simulink model "analog_model_power_v13"  (R2015a)
settings: Solver=ode45  StartTime=0.0  StopTime=12e-3  MaxStep=1e-6  RelTol=1e-3
StartFcn:
  | R1
  | R2
  | R3
  | R4
  | C1
values from neighbouring files (symbols this model uses):
  C = Kp + Ki/s + Kd*s    [DC_Motor_Speed_Digital_Controller_Design_example.m]    (also in GalvoModel_v3_discret_proc.m = gv.tfCCv2p2; InvertedPendulum.m = [1 0 0 0; gtktermFun1.m = textscan(fd, ')
  C2 = 100e-12    (= 1e-10)    [Galvo_sys_proto_v13_OFFSETS_MODEL_PT1B_OLDproc.m]    (also in Galvo_sys_proto_v13_OFFSETS_MODEL_PT1B_proc.m = 1e-11)
  R1 = 1.2e3    (= 1200)    [GalvoModel_v6_sys.m]    (also in Galvo_process_analyze.m = 10000; Galvo_sys_proto_v13_OFFSETS_MODEL_PT1B_OLDproc.m = 5000; Galvo_sys_proto_v13_OFFSETS_MODEL_PT1B_proc.m = 5100; frequenzgang_nichtinvert_opamp_koblitz_eas.m = 0.015)
  R2 = 20e3    (= 20000)    [Galvo_process_analyze.m]    (also in Galvo_sys_proto_v13_OFFSETS_MODEL_PT1B_OLDproc.m = 45000; Galvo_sys_proto_v13_OFFSETS_MODEL_PT1B_proc.m = (Kp-1)*R1; frequenzgang_nichtinvert_opamp_koblitz_eas.m = RL+j*w*L)
  R3 = 1e3    (= 1000)    [Galvo_sys_proto_v13_OFFSETS_MODEL_PT1B_OLDproc.m]    (also in Galvo_sys_proto_v13_OFFSETS_MODEL_PT1B_proc.m = 1e+33)
  R4 = R1    (= 3300)    [Galvo_sys_proto_v13_OFFSETS_MODEL_PT1B_proc.m]    (also in OpAmp_addierer_spannTeiler.m = 10)
  s = tf('s')    [DC_Motor_Speed_Digital_Controller_Design_example.m]    (also in GalvoBIGMatlab_cortex_Link.m = instrfind; GalvoMatlab_cortex_Link.m = MdbOpenPort(); GalvoModel_v6_sys.m; Galvo_process_analyze.m = struct)
undefined symbols (not defined in the file or in its folder): Z4
libraries: fl_lib x24, nesl_utility x6, elec_lib x3, slctrlblks x2, simulink x2
settings Model: Creator=mainster  LastModifiedBy=mainster
settings DebuggingCC: UnderspecifiedInitializationDetection=Classic  MergeDetectMultiDrivingBlocksExec=none  SolverPrmCheckMsg=warning  StateNameClashWarn=warning

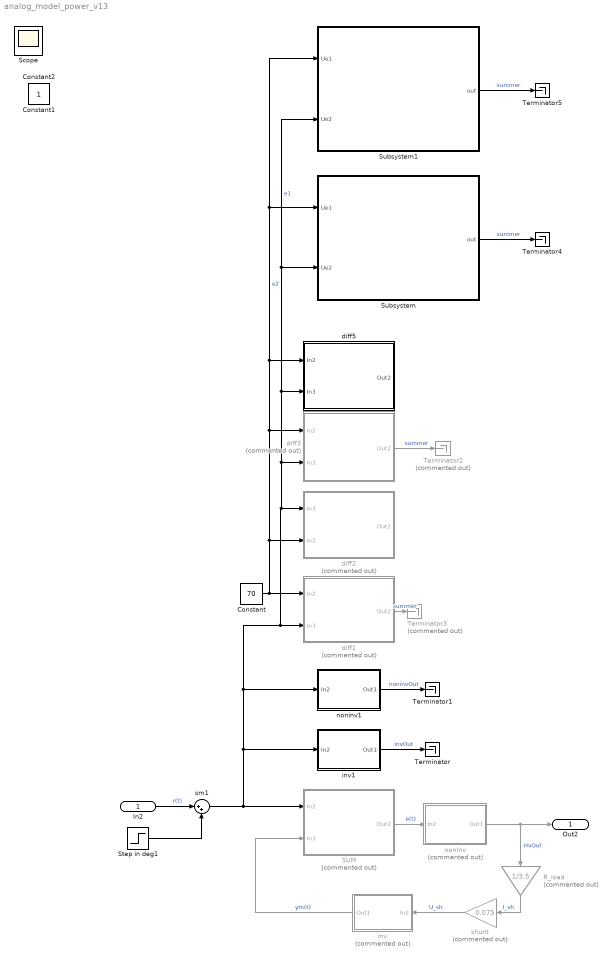
== system analog_model_power_v13 ==
  In2 : Inport
  Constant : Constant  Value=70
  R_load : Gain  Commented=on  Gain=1/3.5
  SUM : Subsystem  Commented=on  mask{R1=3.3e3, R2=3.3e3, R3=3.3e3, R4=3.3e3, C1=1e-12}
      mask prompts: R1 "Value for R1"; R2 "Value for R2"; R3 "Value for R3"; R4 "Value for R4"; C1 "Value for C1"
      mask Display: fprintf('R1=%gohm\nR2=%gohm\nR3=%gohm\nR4=%gohm\nC1=%gnF\n',R1,R2,R3,R4,C1*1e9)
  Step in deg1 : Step  Time=1e-3  SampleTime=0  ZeroCross=off
      settings: AttributesFormatString=Ampl.: %<After>\ntime:%<Time>
  Subsystem : Subsystem  mask{R1=3.3e3, R2=3.3e3, R3=3.3e3, R4=3.3e3}
      mask prompts: R1 "Enter R1"; R2 "Enter R2"; R3 "Enter R3"; R4 "Enter R4"
      mask Display:
      | image(imread('/media/storage/data_notebook/HS_Karlsruhe/xy_galvoscanner/gewichteter_Diff.png'));
      | text(.71, .65, num2str(R4))
      | text(.26, .675, num2str(R3))
      | text(.26, .265, num2str(R1))
      | text(.46, .045, num2str(R2))
  Subsystem1 : Subsystem  mask{R1=3.3e3, R2=3.3e3, R3=3.3e3, R4=3.3e3, C1=100e-12}
      mask prompts: R1 "Enter R1"; R2 "Enter R2"; R3 "Enter R3"; R4 "Enter R4"; C1 "Enter C1"
      mask Callback R4:
      | if C1>0
      |     Z4=R4/(1+s*C1*R4)
      | end
      mask Callback C1:
      | if R4>0
      |     Z4=R4/(1+s*C1*R4)
      | end
      mask Display:
      | image(imread('/media/storage/data_notebook/HS_Karlsruhe/xy_galvoscanner/gewichteter_Diff_lead.png'));
      | text(.71, .65, num2str(R4))
      | text(.26, .675, num2str(R3))
      | text(.26, .265, num2str(R1))
      | text(.46, .045, num2str(R2))
      | text(.76, .842, num2str(R4))
  Terminator{,1,4..5} (4 alike) : Terminator
  Terminator2 : Terminator  Commented=on
  Terminator3 : Terminator  Commented=on
  diff1 : Subsystem  Commented=on  mask{R1=3.3e3, R2=3.3e3, R3=3.3e3, R4=3.3e3, C1=1e-08}
      mask prompts: R1 "Value for R1"; R2 "Value for R2"; R3 "Value for R3"; R4 "Value for R4"; C1 "Value for C1"
      mask Display:
      | fprintf('R1=%gohm\nR2=%gohm\nR3=%gohm\nR4=%gohm\nC1=%gnF\n',R1,R2,R3,R4,C1*1e9)
      | % port_label('input',1,'Ue1');
      | % port_label('input',2,'Ue2');
  diff2 : Subsystem  Commented=on  mask{R1=3.3e3, R2=3.3e3, R3=3.3e3, R4=3.3e3, C1=1e-11}
      mask prompts: R1 "Value for R1"; R2 "Value for R2"; R3 "Value for R3"; R4 "Value for R4"; C1 "Value for C1"
      mask Display:
      | fprintf('R1=%gohm\nR2=%gohm\nR3=%gohm\nR4=%gohm\nC1=%gnF\n',R1,R2,R3,R4,C1*1e9)
      | % port_label('input',1,'Ue1');
      | % port_label('input',2,'Ue2');
  diff3 : Subsystem  Commented=on  mask{R1=3e3, gR1=1/R1, R2=3e3, gR2=1/R2, R3=3e3, R4=3e3, R4R3=R4/R3, C1=1e-11, gC1=0, C2=1e-35, gC2=1/C2}
      mask prompts: R1 "Value for R1"; gR1 "Gain:"; R2 "Value for R2"; gR2 "Gain:"; R3 "Value for R3"; R4 "Value for R4"; R4R3 "Gain:"; C1 "Value for C1"; C2 "Value for C2"; gC2 "Gain:"
      mask Callback R1: gR1=1/R1
      mask TypeOptions gR1: Gain3/Gain
      mask Callback R2: gR2=1/R2
      mask TypeOptions gR2: Gain1/Gain
      mask Callback R3:
      | if R3>0
      |     R4R3 = R4/R3;
      | end
      mask Callback R4:
      | if R3>0
      |     R4R3 = R4/R3;
      | end
      mask TypeOptions R4R3: Gain4/Gain
      mask Callback C1: gC1=1/C1
      mask Callback C2: gC2=1/C2
      mask TypeOptions gC2: Gain/Gain
      mask Display:
      | fprintf('R1=%gohm\nR2=%gohm\nR3=%gohm\nR4=%gohm\nC1=%gF\nC2=%gF\n',R1,R2,R3,R4,C1,C2)
      | % port_label('input',1,'Ue1');
      | % port_label('input',2,'Ue2');
  diff5 : Subsystem  mask{R1=3.3e3, R2=3.3e3, R3=3.3e3, R4=3.3e3, C1=1e-11, C2=1}
      mask prompts: R1 "Value for R1"; R2 "Value for R2"; R3 "Value for R3"; R4 "Value for R4"; C1 "Value for C1"; C2 "Value for C2"
      mask Display:
      | fprintf('R1=%gohm\nR2=%gohm\nR3=%gohm\nR4=%gohm\nC1=%gnF\n',R1,R2,R3,R4,C1*1e9)
      | % port_label('input',1,'Ue1');
      | % port_label('input',2,'Ue2');
  inv : Subsystem  Commented=on  mask{R1=27, R2=270, C1=1}
      mask prompts: R1 "Value for R1"; R2 "Value for R2"; C1 "Value for C1"
      mask Display: fprintf('R1=%gohm\nR2=%gohm\nC1=%gnF\n',R1,R2,C1*1e9)
  inv1 : Subsystem  mask{R1=1e3, R2=10e3, C2=1e-11}
      mask prompts: R1 "Value for R1"; R2 "Value for R2"; C2 "Value for C2"
      mask Display: fprintf('R1=%gohm\nR2=%gohm\nC2=%gF\n',R1,R2,C2)
  nonInv : Subsystem  Commented=on  mask{R1=5.1e3, R2=2*5.1e3, C2=1e-08}
      mask prompts: R1 "Value for R1"; R2 "Value for R2"; C2 "Value for C2"
      mask Display: fprintf('R1=%gohm\nR2=%gohm\nC1=C2=%gF\n',R1,R2,C2)
  noninv1 : Subsystem  mask{R1=1e3, R2=9e3, C2=1e-08}
      mask prompts: R1 "Value for R1"; R2 "Value for R2"; C2 "Value for C2"
      mask Display: fprintf('R1=%gohm\nR2=%gohm\nC2=%gF\n',R1,R2,C2)
  shunt : Gain  Commented=on  Gain=0.075
  sm1 : Sum  Inputs=|++
  Out2 : Outport
  Constant1 : Constant  IOType=siggen
  Constant2 : Constant  IOType=siggen
  Scope : Scope  NumInputPorts=4
      settings: ShowLegends=on  TimeRange=0.012  YMin=-5~-5~-5~-5  YMax=5~5~5~5  MaxDataPoints=7500
  wires:
  SUM/1(Out2) -> nonInv/1(In2)  "e(t)"
  In2/1 -> sm1/1  "r(t)"
  inv/1(Out1) -> SUM/2(In3)  "ym(t)"
  nonInv/1(Out1) -> R_load/1, Out2/1  "HvOut"
  R_load/1 -> shunt/1  "I_sh"
  shunt/1 -> inv/1(In2)  "U_sh"
  Step in deg1/1 -> sm1/2
  inv1/1(Out1) -> Terminator/1  "invOut"
  noninv1/1(Out1) -> Terminator1/1  "noninvOut"
  diff3/1(Out2) -> Terminator2/1  "summer"
  diff1/1(Out2) -> Terminator3/1  "summer"
  Subsystem/1(out) -> Terminator4/1  "summer"
  sm1/1 -> Subsystem1/2(Ue2), Subsystem/2(Ue2), diff5/2(In3), diff3/2(In3), diff2/1(In3), diff1/2(In3), noninv1/1(In2), inv1/1(In2), SUM/1(In2)  "e1"
  Constant/1 -> Subsystem1/1(Ue1), Subsystem/1(Ue1), diff5/1(In2), diff3/1(In2), diff2/2(In2), diff1/1(In2)  "e2"
  Subsystem1/1(out) -> Terminator5/1  "summer"

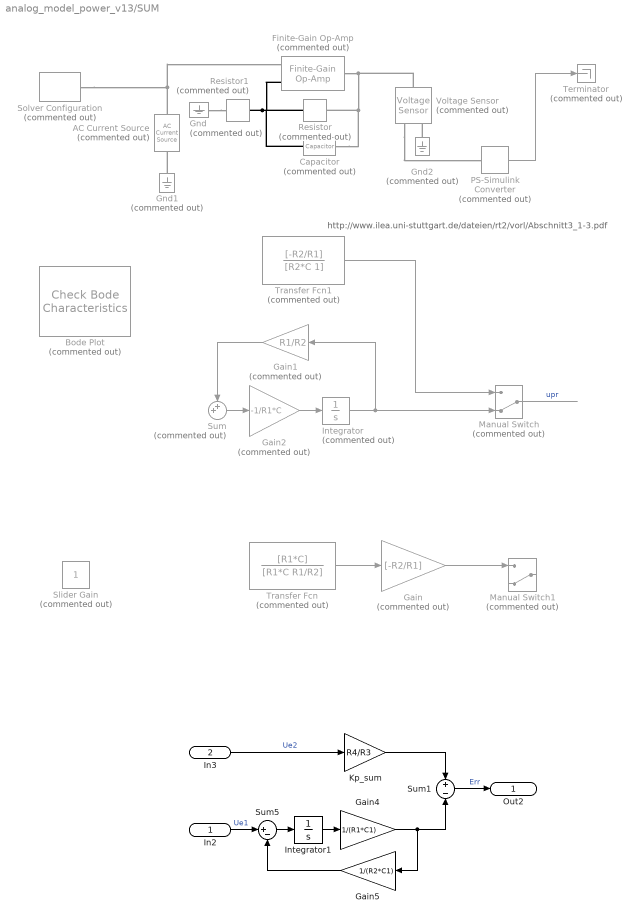
== system analog_model_power_v13/SUM ==
  note: http://www.ilea.uni-stuttgart.de/dateien/rt2/vorl/Abschnitt3_1-3.pdf
  In2 : Inport
  In3 : Inport  Port=2
  AC Current Source : fl_lib/Electrical/Electrical Sources/AC Current Source  Commented=on  amp=1 A  shift=0 deg  frequency=1000 Hz  omega=0 rad/s  i_Log=off  v_Log=off  LocalVarNames=|i|v  LocalVarDescs=|i|v  LocalVarLogging=[0 0]
  Bode Plot : slctrlblks/Model Verification/Check Bode  Characteristics  Commented=on  InstantiateOnLoad=on  SaveOperatingPoints=off  LinearizationIOs={'/Gcc(s)/sub1/In1', 1, 'in', 'off', '';'/Gcc(s)/sub1/Gain', 1, 'out', 'on', '';'/Gcc(s)/sub1/Manual Switch', 1, 'out', 'on', '';'/Gcc(s)/sub1/Manual Switch1', 1, 'out', 'on', ''}  LinearizeAt=SnapshotTimes  SnapshotTimes=[0]  TriggerType=rising  SampleTime=auto  RateConversionMethod=zoh  PreWarpFreq=10  UseExactDelayModel=off  UseFullBlockNameLabels=off  UseBusSignalLabels=off  enabled=on  stopWhenAssertionFail=off  export=off  ViewDlgPos=[100 200 510 390]  OpenViewOnLoad=off  LaunchViewOnOpen=on  FrequencyUnits=rad/s  MagnitudeUnits=dB  PhaseUnits=deg  TimeUnits=seconds  EnableUpperBound=off  UpperBoundFrequencies=[]  UpperBoundMagnitudes=[]  EnableLowerBound=off  LowerBoundFrequencies=[]  LowerBoundMagnitudes=[]
  Capacitor : fl_lib/Electrical/Electrical Elements/Capacitor  Commented=on  c=1e-6 F  v0=0 V  r=1e-6 Ohm  g=0 1/Ohm  i_Log=off  v_Log=off  vc_Log=off  LocalVarNames=|i|v|vc  LocalVarDescs=|i|v|Internal variable for voltage across capacitor term  LocalVarLogging=[0 0 0]
  Finite-Gain Op-Amp : elec_lib/Integrated Circuits/Finite-Gain Op-Amp  Commented=on  A=1000  Rin=1e+6 Ohm  Rout=100 Ohm  Vmin=-15 V  Vmax=15 V  LocalVarLogging=[]
  Gain : Gain  Commented=on  Gain=[-R2/R1]
  Gain1 : Gain  Commented=on  Gain=R1/R2
  Gain2 : Gain  Commented=on  Gain=-1/R1*C
  Gain4 : Gain  Gain=1/(R1*C1)
  Gain5 : Gain  Gain=1/(R2*C1)
  Gnd : fl_lib/Electrical/Electrical Elements/Electrical Reference  Commented=on  i_Log=off  LocalVarNames=|i  LocalVarDescs=|i  LocalVarLogging=0
  Gnd1 : fl_lib/Electrical/Electrical Elements/Electrical Reference  Commented=on  i_Log=off  LocalVarNames=|i  LocalVarDescs=|i  LocalVarLogging=0
  Gnd2 : fl_lib/Electrical/Electrical Elements/Electrical Reference  Commented=on  i_Log=off  LocalVarNames=|i  LocalVarDescs=|i  LocalVarLogging=0
  Integrator : Integrator  Commented=on
  Integrator1 : Integrator
  Kp_sum : Gain  Gain=R4/R3
  Manual Switch : ManualSwitch  Commented=on  CurrentSetting=0
  Manual Switch1 : ManualSwitch  Commented=on  CurrentSetting=0
  PS-Simulink Converter : nesl_utility/PS-Simulink Converter  Commented=on  PhysicalDomain=network_engine_domain  SubClassName=ps_output  LeftPortType=input  RightPortType=output  PseudoPeriodic=off  Frequencies=[]  Unit=1  AffineConversion=off
  Resistor : fl_lib/Electrical/Electrical Elements/Resistor  Commented=on  R=R2 Ohm  i_Log=off  v_Log=off  LocalVarNames=|i|v  LocalVarDescs=|i|v  LocalVarLogging=[0 0]
      settings: AttributesFormatString=%<R>
  Resistor1 : fl_lib/Electrical/Electrical Elements/Resistor  Commented=on  R=R1 Ohm  i_Log=off  v_Log=off  LocalVarNames=|i|v  LocalVarDescs=|i|v  LocalVarLogging=[0 0]
      settings: AttributesFormatString=%<R>
  Slider Gain : simulink/Math Operations/Slider Gain  Commented=on  low=0  gain=1  high=2
  Solver Configuration : nesl_utility/Solver Configuration  Commented=on  PhysicalDomain=network_engine_domain  SubClassName=solver  LeftPortType=input  RightPortType=generic  Accelerate=off  Tones=[]  Harmonics=[]  SimulateNoise=off  Profile=off  UseLocalSampling=off  EnableSwitchedLinearOptims=on  FrequencyDomain=off  UseCCode=off  UseNewInitialization=off  DoDC=off  ResidualTolerance=1e-09  UseLocalSolver=off  LocalSolverChoice=NE_BACKWARD_EULER_ADVANCER  LocalSolverSampleTime=0.001  DoFixedCost=off  MaxNonlinIter=3  MaxModeIter=2  LinearAlgebra=Sparse  DelaysMemoryBudget=1024
  Sum : Sum  Commented=on  Inputs=++|
  Sum1 : Sum  Inputs=+|-
  Sum5 : Sum  Inputs=|+-
  Terminator : Terminator  Commented=on
  Transfer Fcn : TransferFcn  Commented=on  Numerator=[R1*C]  Denominator=[R1*C R1/R2]
  Transfer Fcn1 : TransferFcn  Commented=on  Numerator=[-R2/R1]  Denominator=[R2*C 1]
  Voltage Sensor : fl_lib/Electrical/Electrical Sensors/Voltage Sensor  Commented=on  i1_Log=off  v1_Log=off  LocalVarNames=|i1|v1  LocalVarDescs=|i1|v1  LocalVarLogging=[0 0]
  Out2 : Outport
  wires:
  Integrator1/1 -> Gain4/1
  Gain4/1 -> Gain5/1, Sum1/2
  ? -> Transfer Fcn/1, Transfer Fcn1/1, Sum/2
  Transfer Fcn/1 -> Gain/1
  Sum5/1 -> Integrator1/1
  Manual Switch/1 -> ?  "upr"
  Gain/1 -> Manual Switch1/1
  Gain1/1 -> Sum/1
  Integrator/1 -> Gain1/1, Manual Switch/2
  Sum/1 -> Gain2/1
  Gain2/1 -> Integrator/1
  Transfer Fcn1/1 -> Manual Switch/1
  PS-Simulink Converter/1 -> Terminator/1
  Gain5/1 -> Sum5/2
  In3/1 -> Kp_sum/1  "Ue2"
  Kp_sum/1 -> Sum1/1
  In2/1 -> Sum5/1  "Ue1"
  Sum1/1 -> Out2/1  "Err"
  connections:
  Resistor1/RConn1 -- Capacitor/LConn1 -- Finite-Gain Op-Amp/LConn2 -- Resistor/LConn1
  Solver Configuration/RConn1 -- Finite-Gain Op-Amp/LConn1 -- AC Current Source/LConn1
  Gnd1/LConn1 -- AC Current Source/RConn1
  Voltage Sensor/RConn1 -- PS-Simulink Converter/LConn1
  Gnd2/LConn1 -- Voltage Sensor/RConn2
  Gnd/LConn1 -- Resistor1/LConn1
  Voltage Sensor/LConn1 -- Capacitor/RConn1 -- Resistor/RConn1 -- Finite-Gain Op-Amp/RConn1

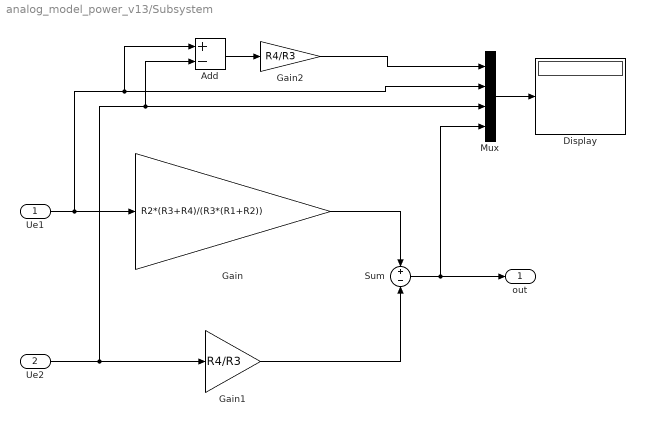
== system analog_model_power_v13/Subsystem ==
  Ue1 : Inport
  Ue2 : Inport  Port=2
  Add : Sum  Inputs=+-
  Display : Display
  Gain : Gain  Gain=R2*(R3+R4)/(R3*(R1+R2))
  Gain1 : Gain  Gain=R4/R3
  Gain2 : Gain  Gain=R4/R3
  Mux : Mux
  Sum : Sum  Inputs=+|-
  out : Outport
  wires:
  Gain/1 -> Sum/1
  Gain1/1 -> Sum/2
  Ue1/1 -> Mux/2, Add/1, Gain/1
  Ue2/1 -> Mux/3, Add/2, Gain1/1
  Sum/1 -> Mux/4, out/1
  Mux/1 -> Display/1
  Add/1 -> Gain2/1
  Gain2/1 -> Mux/1

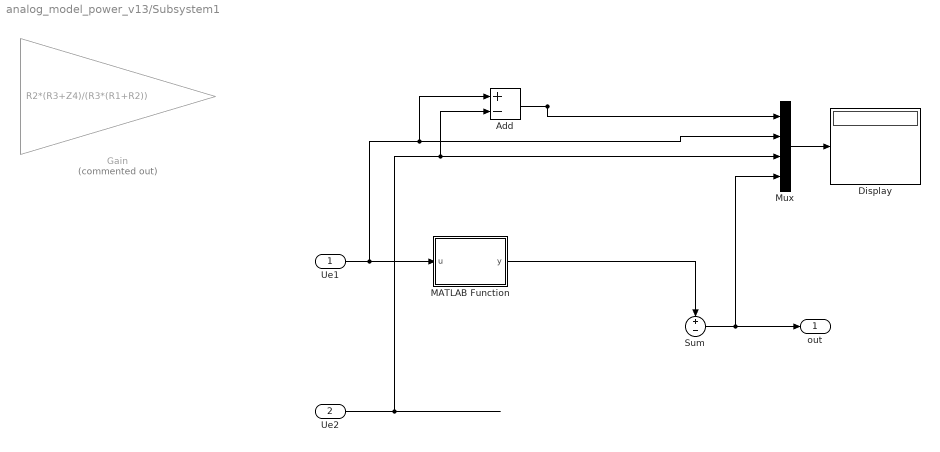
== system analog_model_power_v13/Subsystem1 ==
  Ue1 : Inport
  Ue2 : Inport  Port=2
  Add : Sum  Inputs=+-
  Display : Display
  Gain : Gain  Commented=on  Gain=R2*(R3+Z4)/(R3*(R1+R2))
  MATLAB Function : MATLAB Function  TreatAsAtomicUnit=on
  Mux : Mux
  Sum : Sum  Inputs=+|-
  out : Outport
  wires:
  MATLAB Function/1(y) -> Sum/1
  ? -> Sum/2
  Ue1/1 -> MATLAB Function/1(u), Mux/2, Add/1
  Ue2/1 -> Mux/3, Add/2
  Sum/1 -> Mux/4, out/1
  Mux/1 -> Display/1
  Add/1 -> Mux/1

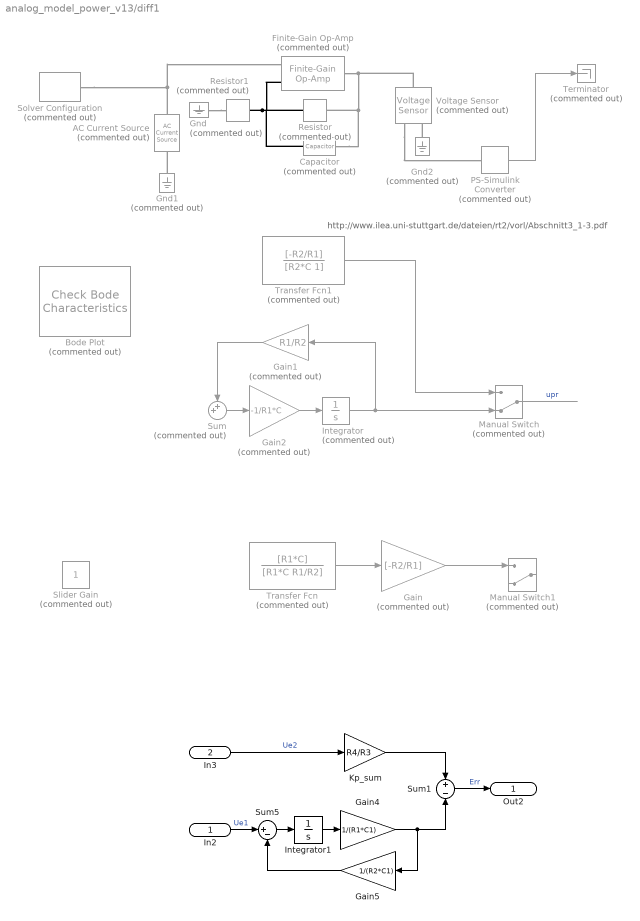
== system analog_model_power_v13/diff1 ==
  note: http://www.ilea.uni-stuttgart.de/dateien/rt2/vorl/Abschnitt3_1-3.pdf
  In2 : Inport
  In3 : Inport  Port=2
  AC Current Source : fl_lib/Electrical/Electrical Sources/AC Current Source  Commented=on  amp=1 A  shift=0 deg  frequency=1000 Hz  omega=0 rad/s  i_Log=off  v_Log=off  LocalVarNames=|i|v  LocalVarDescs=|i|v  LocalVarLogging=[0 0]
  Bode Plot : slctrlblks/Model Verification/Check Bode  Characteristics  Commented=on  InstantiateOnLoad=on  SaveOperatingPoints=off  LinearizationIOs={'/Gcc(s)/sub1/In1', 1, 'in', 'off', '';'/Gcc(s)/sub1/Gain', 1, 'out', 'on', '';'/Gcc(s)/sub1/Manual Switch', 1, 'out', 'on', '';'/Gcc(s)/sub1/Manual Switch1', 1, 'out', 'on', ''}  LinearizeAt=SnapshotTimes  SnapshotTimes=[0]  TriggerType=rising  SampleTime=auto  RateConversionMethod=zoh  PreWarpFreq=10  UseExactDelayModel=off  UseFullBlockNameLabels=off  UseBusSignalLabels=off  enabled=on  stopWhenAssertionFail=off  export=off  ViewDlgPos=[100 200 510 390]  OpenViewOnLoad=off  LaunchViewOnOpen=on  FrequencyUnits=rad/s  MagnitudeUnits=dB  PhaseUnits=deg  TimeUnits=seconds  EnableUpperBound=off  UpperBoundFrequencies=[]  UpperBoundMagnitudes=[]  EnableLowerBound=off  LowerBoundFrequencies=[]  LowerBoundMagnitudes=[]
  Capacitor : fl_lib/Electrical/Electrical Elements/Capacitor  Commented=on  c=1e-6 F  v0=0 V  r=1e-6 Ohm  g=0 1/Ohm  i_Log=off  v_Log=off  vc_Log=off  LocalVarNames=|i|v|vc  LocalVarDescs=|i|v|Internal variable for voltage across capacitor term  LocalVarLogging=[0 0 0]
  Finite-Gain Op-Amp : elec_lib/Integrated Circuits/Finite-Gain Op-Amp  Commented=on  A=1000  Rin=1e+6 Ohm  Rout=100 Ohm  Vmin=-15 V  Vmax=15 V  LocalVarLogging=[]
  Gain : Gain  Commented=on  Gain=[-R2/R1]
  Gain1 : Gain  Commented=on  Gain=R1/R2
  Gain2 : Gain  Commented=on  Gain=-1/R1*C
  Gain4 : Gain  Gain=1/(R1*C1)
  Gain5 : Gain  Gain=1/(R2*C1)
  Gnd : fl_lib/Electrical/Electrical Elements/Electrical Reference  Commented=on  i_Log=off  LocalVarNames=|i  LocalVarDescs=|i  LocalVarLogging=0
  Gnd1 : fl_lib/Electrical/Electrical Elements/Electrical Reference  Commented=on  i_Log=off  LocalVarNames=|i  LocalVarDescs=|i  LocalVarLogging=0
  Gnd2 : fl_lib/Electrical/Electrical Elements/Electrical Reference  Commented=on  i_Log=off  LocalVarNames=|i  LocalVarDescs=|i  LocalVarLogging=0
  Integrator : Integrator  Commented=on
  Integrator1 : Integrator
  Kp_sum : Gain  Gain=R4/R3
  Manual Switch : ManualSwitch  Commented=on  CurrentSetting=0
  Manual Switch1 : ManualSwitch  Commented=on  CurrentSetting=0
  PS-Simulink Converter : nesl_utility/PS-Simulink Converter  Commented=on  PhysicalDomain=network_engine_domain  SubClassName=ps_output  LeftPortType=input  RightPortType=output  PseudoPeriodic=off  Frequencies=[]  Unit=1  AffineConversion=off
  Resistor : fl_lib/Electrical/Electrical Elements/Resistor  Commented=on  R=R2 Ohm  i_Log=off  v_Log=off  LocalVarNames=|i|v  LocalVarDescs=|i|v  LocalVarLogging=[0 0]
      settings: AttributesFormatString=%<R>
  Resistor1 : fl_lib/Electrical/Electrical Elements/Resistor  Commented=on  R=R1 Ohm  i_Log=off  v_Log=off  LocalVarNames=|i|v  LocalVarDescs=|i|v  LocalVarLogging=[0 0]
      settings: AttributesFormatString=%<R>
  Slider Gain : simulink/Math Operations/Slider Gain  Commented=on  low=0  gain=1  high=2
  Solver Configuration : nesl_utility/Solver Configuration  Commented=on  PhysicalDomain=network_engine_domain  SubClassName=solver  LeftPortType=input  RightPortType=generic  Accelerate=off  Tones=[]  Harmonics=[]  SimulateNoise=off  Profile=off  UseLocalSampling=off  EnableSwitchedLinearOptims=on  FrequencyDomain=off  UseCCode=off  UseNewInitialization=off  DoDC=off  ResidualTolerance=1e-09  UseLocalSolver=off  LocalSolverChoice=NE_BACKWARD_EULER_ADVANCER  LocalSolverSampleTime=0.001  DoFixedCost=off  MaxNonlinIter=3  MaxModeIter=2  LinearAlgebra=Sparse  DelaysMemoryBudget=1024
  Sum : Sum  Commented=on  Inputs=++|
  Sum1 : Sum  Inputs=+|-
  Sum5 : Sum  Inputs=|+-
  Terminator : Terminator  Commented=on
  Transfer Fcn : TransferFcn  Commented=on  Numerator=[R1*C]  Denominator=[R1*C R1/R2]
  Transfer Fcn1 : TransferFcn  Commented=on  Numerator=[-R2/R1]  Denominator=[R2*C 1]
  Voltage Sensor : fl_lib/Electrical/Electrical Sensors/Voltage Sensor  Commented=on  i1_Log=off  v1_Log=off  LocalVarNames=|i1|v1  LocalVarDescs=|i1|v1  LocalVarLogging=[0 0]
  Out2 : Outport
  wires:
  Integrator1/1 -> Gain4/1
  Gain4/1 -> Gain5/1, Sum1/2
  ? -> Transfer Fcn/1, Transfer Fcn1/1, Sum/2
  Transfer Fcn/1 -> Gain/1
  Sum5/1 -> Integrator1/1
  Manual Switch/1 -> ?  "upr"
  Gain/1 -> Manual Switch1/1
  Gain1/1 -> Sum/1
  Integrator/1 -> Gain1/1, Manual Switch/2
  Sum/1 -> Gain2/1
  Gain2/1 -> Integrator/1
  Transfer Fcn1/1 -> Manual Switch/1
  PS-Simulink Converter/1 -> Terminator/1
  Gain5/1 -> Sum5/2
  In3/1 -> Kp_sum/1  "Ue2"
  Kp_sum/1 -> Sum1/1
  In2/1 -> Sum5/1  "Ue1"
  Sum1/1 -> Out2/1  "Err"
  connections:
  Resistor1/RConn1 -- Capacitor/LConn1 -- Finite-Gain Op-Amp/LConn2 -- Resistor/LConn1
  Solver Configuration/RConn1 -- Finite-Gain Op-Amp/LConn1 -- AC Current Source/LConn1
  Gnd1/LConn1 -- AC Current Source/RConn1
  Voltage Sensor/RConn1 -- PS-Simulink Converter/LConn1
  Gnd2/LConn1 -- Voltage Sensor/RConn2
  Gnd/LConn1 -- Resistor1/LConn1
  Voltage Sensor/LConn1 -- Capacitor/RConn1 -- Resistor/RConn1 -- Finite-Gain Op-Amp/RConn1

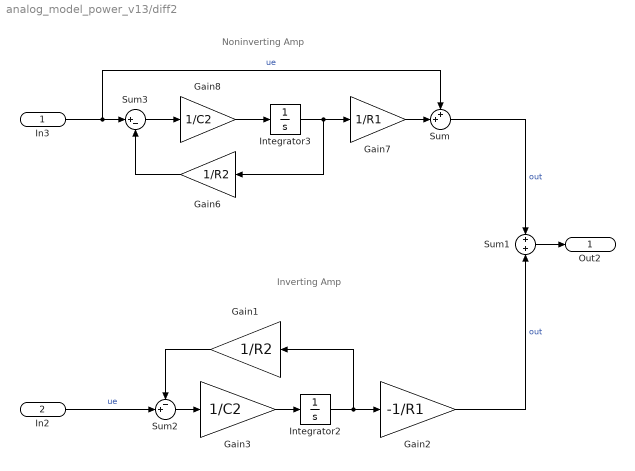
== system analog_model_power_v13/diff2 ==
  note: Inverting Amp
  note: Noninverting Amp
  In3 : Inport
  In2 : Inport  Port=2
  Gain1 : Gain  Gain=1/R2
  Gain2 : Gain  Gain=-1/R1
  Gain3 : Gain  Gain=1/C2
  Gain6 : Gain  Gain=1/R2
  Gain7 : Gain  Gain=1/R1
  Gain8 : Gain  Gain=1/C2
  Integrator2 : Integrator
  Integrator3 : Integrator
  Sum : Sum  Inputs=++|
  Sum1 : Sum  Inputs=+|+
  Sum2 : Sum  Inputs=-+|
  Sum3 : Sum  Inputs=|+-
  Out2 : Outport
  wires:
  Integrator2/1 -> Gain1/1, Gain2/1
  In2/1 -> Sum2/2  "ue"
  Gain3/1 -> Integrator2/1
  Gain2/1 -> Sum1/2  "out"
  Sum2/1 -> Gain3/1
  Gain1/1 -> Sum2/1
  Integrator3/1 -> Gain6/1, Gain7/1
  In3/1 -> Sum/1, Sum3/1  "ue"
  Gain8/1 -> Integrator3/1
  Sum/1 -> Sum1/1  "out"
  Sum3/1 -> Gain8/1
  Gain6/1 -> Sum3/2
  Gain7/1 -> Sum/2
  Sum1/1 -> Out2/1

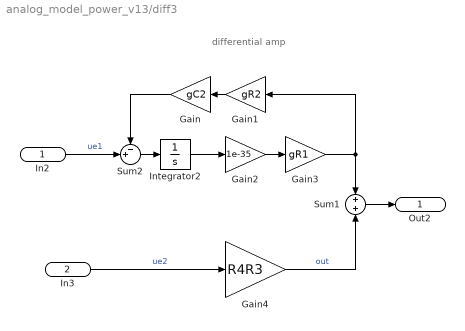
== system analog_model_power_v13/diff3 ==
  note: differential amp
  In2 : Inport
  In3 : Inport  Port=2
  Gain : Gain  Gain=gC2
  Gain1 : Gain  Gain=gR2
  Gain2 : Gain  Gain=1e-35
  Gain3 : Gain  Gain=gR1
  Gain4 : Gain  Gain=R4R3
  Integrator2 : Integrator
  Sum1 : Sum  Inputs=+|+
  Sum2 : Sum  Inputs=-+|
  Out2 : Outport
  wires:
  In2/1 -> Sum2/2  "ue1"
  In3/1 -> Gain4/1  "ue2"
  Sum2/1 -> Integrator2/1
  Gain/1 -> Sum2/1
  Gain4/1 -> Sum1/2  "out"
  Sum1/1 -> Out2/1
  Gain1/1 -> Gain/1
  Integrator2/1 -> Gain2/1
  Gain2/1 -> Gain3/1
  Gain3/1 -> Gain1/1, Sum1/1

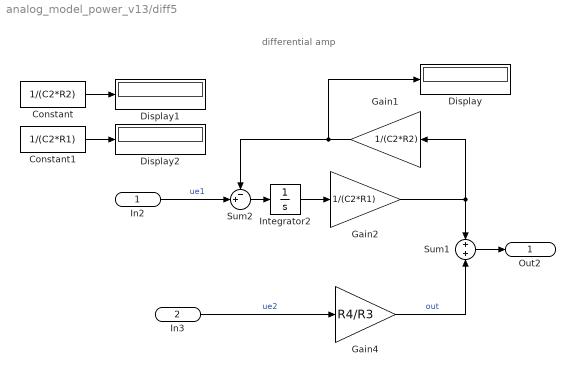
== system analog_model_power_v13/diff5 ==
  note: differential amp
  In2 : Inport
  In3 : Inport  Port=2
  Constant : Constant  Value=1/(C2*R2)
  Constant1 : Constant  Value=1/(C2*R1)
  Display : Display
  Display1 : Display
  Display2 : Display
  Gain1 : Gain  Gain=1/(C2*R2)
  Gain2 : Gain  Gain=1/(C2*R1)
  Gain4 : Gain  Gain=R4/R3
  Integrator2 : Integrator
  Sum1 : Sum  Inputs=+|+
  Sum2 : Sum  Inputs=-+|
  Out2 : Outport
  wires:
  In2/1 -> Sum2/2  "ue1"
  In3/1 -> Gain4/1  "ue2"
  Sum2/1 -> Integrator2/1
  Gain1/1 -> Display/1, Sum2/1
  Gain4/1 -> Sum1/2  "out"
  Sum1/1 -> Out2/1
  Gain2/1 -> Gain1/1, Sum1/1
  Integrator2/1 -> Gain2/1
  Constant/1 -> Display1/1
  Constant1/1 -> Display2/1

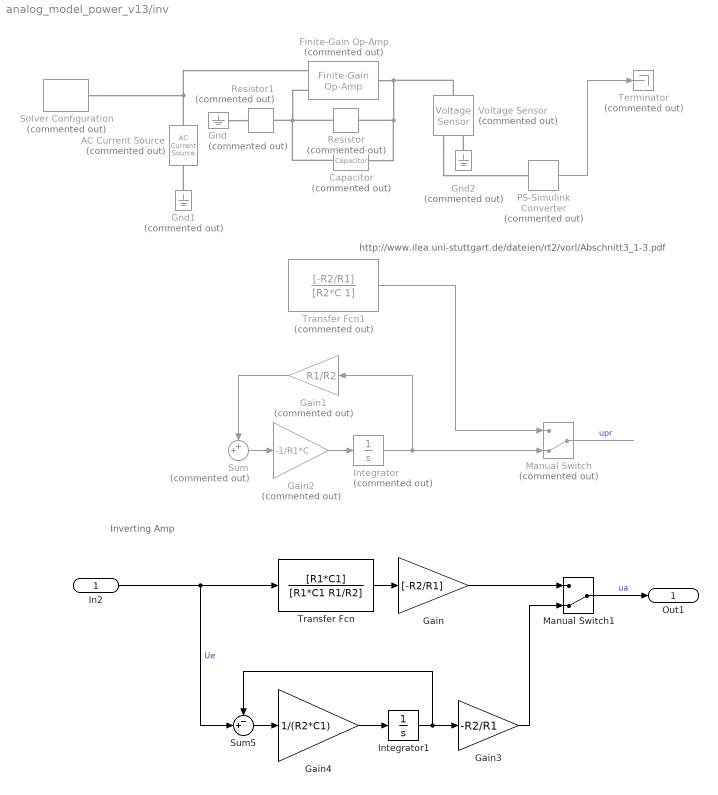
== system analog_model_power_v13/inv ==
  note: Inverting Amp
  note: http://www.ilea.uni-stuttgart.de/dateien/rt2/vorl/Abschnitt3_1-3.pdf
  In2 : Inport
  AC Current Source : fl_lib/Electrical/Electrical Sources/AC Current Source  Commented=on  amp=1 A  shift=0 deg  frequency=1000 Hz  omega=0 rad/s  i_Log=off  v_Log=off  LocalVarNames=|i|v  LocalVarDescs=|i|v  LocalVarLogging=[0 0]
  Capacitor : fl_lib/Electrical/Electrical Elements/Capacitor  Commented=on  c=1e-6 F  v0=0 V  r=1e-6 Ohm  g=0 1/Ohm  i_Log=off  v_Log=off  vc_Log=off  LocalVarNames=|i|v|vc  LocalVarDescs=|i|v|Internal variable for voltage across capacitor term  LocalVarLogging=[0 0 0]
  Finite-Gain Op-Amp : elec_lib/Integrated Circuits/Finite-Gain Op-Amp  Commented=on  A=1000  Rin=1e+6 Ohm  Rout=100 Ohm  Vmin=-15 V  Vmax=15 V  LocalVarLogging=[]
  Gain : Gain  Gain=[-R2/R1]
  Gain1 : Gain  Commented=on  Gain=R1/R2
  Gain2 : Gain  Commented=on  Gain=-1/R1*C
  Gain3 : Gain  Gain=-R2/R1
  Gain4 : Gain  Gain=1/(R2*C1)
  Gnd : fl_lib/Electrical/Electrical Elements/Electrical Reference  Commented=on  i_Log=off  LocalVarNames=|i  LocalVarDescs=|i  LocalVarLogging=0
  Gnd1 : fl_lib/Electrical/Electrical Elements/Electrical Reference  Commented=on  i_Log=off  LocalVarNames=|i  LocalVarDescs=|i  LocalVarLogging=0
  Gnd2 : fl_lib/Electrical/Electrical Elements/Electrical Reference  Commented=on  i_Log=off  LocalVarNames=|i  LocalVarDescs=|i  LocalVarLogging=0
  Integrator : Integrator  Commented=on
  Integrator1 : Integrator
  Manual Switch : ManualSwitch  Commented=on  CurrentSetting=0
  Manual Switch1 : ManualSwitch  CurrentSetting=0
  PS-Simulink Converter : nesl_utility/PS-Simulink Converter  Commented=on  PhysicalDomain=network_engine_domain  SubClassName=ps_output  LeftPortType=input  RightPortType=output  PseudoPeriodic=off  Frequencies=[]  Unit=1  AffineConversion=off
  Resistor : fl_lib/Electrical/Electrical Elements/Resistor  Commented=on  R=R2 Ohm  i_Log=off  v_Log=off  LocalVarNames=|i|v  LocalVarDescs=|i|v  LocalVarLogging=[0 0]
      settings: AttributesFormatString=%<R>
  Resistor1 : fl_lib/Electrical/Electrical Elements/Resistor  Commented=on  R=R1 Ohm  i_Log=off  v_Log=off  LocalVarNames=|i|v  LocalVarDescs=|i|v  LocalVarLogging=[0 0]
      settings: AttributesFormatString=%<R>
  Solver Configuration : nesl_utility/Solver Configuration  Commented=on  PhysicalDomain=network_engine_domain  SubClassName=solver  LeftPortType=input  RightPortType=generic  Accelerate=off  Tones=[]  Harmonics=[]  SimulateNoise=off  Profile=off  UseLocalSampling=off  EnableSwitchedLinearOptims=on  FrequencyDomain=off  UseCCode=off  UseNewInitialization=off  DoDC=off  ResidualTolerance=1e-09  UseLocalSolver=off  LocalSolverChoice=NE_BACKWARD_EULER_ADVANCER  LocalSolverSampleTime=0.001  DoFixedCost=off  MaxNonlinIter=3  MaxModeIter=2  LinearAlgebra=Sparse  DelaysMemoryBudget=1024
  Sum : Sum  Commented=on  Inputs=++|
  Sum5 : Sum  Inputs=-+|
  Terminator : Terminator  Commented=on
  Transfer Fcn : TransferFcn  Numerator=[R1*C1]  Denominator=[R1*C1 R1/R2]
  Transfer Fcn1 : TransferFcn  Commented=on  Numerator=[-R2/R1]  Denominator=[R2*C 1]
  Voltage Sensor : fl_lib/Electrical/Electrical Sensors/Voltage Sensor  Commented=on  i1_Log=off  v1_Log=off  LocalVarNames=|i1|v1  LocalVarDescs=|i1|v1  LocalVarLogging=[0 0]
  Out1 : Outport
  wires:
  Integrator1/1 -> Gain3/1, Sum5/1
  Gain3/1 -> Manual Switch1/2
  In2/1 -> Transfer Fcn/1, Sum5/2  "Ue"
  Transfer Fcn/1 -> Gain/1
  Gain4/1 -> Integrator1/1
  Gain/1 -> Manual Switch1/1
  Manual Switch1/1 -> Out1/1  "ua"
  Sum5/1 -> Gain4/1
  Manual Switch/1 -> ?  "upr"
  Gain1/1 -> Sum/1
  Integrator/1 -> Gain1/1, Manual Switch/2
  Sum/1 -> Gain2/1
  Gain2/1 -> Integrator/1
  Transfer Fcn1/1 -> Manual Switch/1
  PS-Simulink Converter/1 -> Terminator/1
  connections:
  Capacitor/LConn1 -- Resistor1/RConn1 -- Finite-Gain Op-Amp/LConn2 -- Resistor/LConn1
  Solver Configuration/RConn1 -- Finite-Gain Op-Amp/LConn1 -- AC Current Source/LConn1
  Finite-Gain Op-Amp/RConn1 -- Voltage Sensor/LConn1 -- Resistor/RConn1 -- Capacitor/RConn1
  Gnd1/LConn1 -- AC Current Source/RConn1
  Gnd/LConn1 -- Resistor1/LConn1
  Voltage Sensor/RConn1 -- PS-Simulink Converter/LConn1
  Gnd2/LConn1 -- Voltage Sensor/RConn2

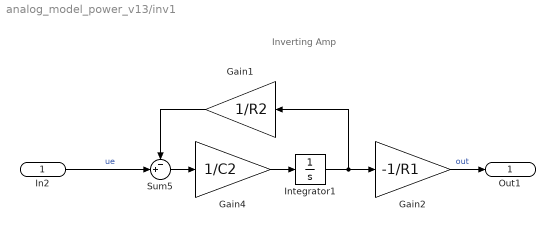
== system analog_model_power_v13/inv1 ==
  note: Inverting Amp
  In2 : Inport
  Gain1 : Gain  Gain=1/R2
  Gain2 : Gain  Gain=-1/R1
  Gain4 : Gain  Gain=1/C2
  Integrator1 : Integrator
  Sum5 : Sum  Inputs=-+|
  Out1 : Outport
  wires:
  Integrator1/1 -> Gain1/1, Gain2/1
  In2/1 -> Sum5/2  "ue"
  Gain4/1 -> Integrator1/1
  Gain2/1 -> Out1/1  "out"
  Sum5/1 -> Gain4/1
  Gain1/1 -> Sum5/1

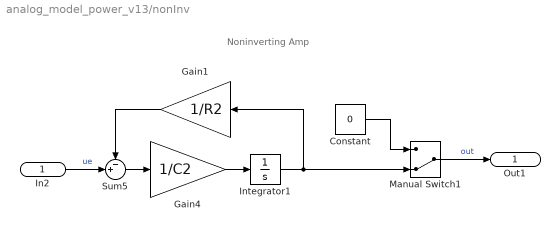
== system analog_model_power_v13/nonInv ==
  note: Noninverting Amp
  In2 : Inport
  Constant : Constant  Value=0
  Gain1 : Gain  Gain=1/R2
  Gain4 : Gain  Gain=1/C2
  Integrator1 : Integrator
  Manual Switch1 : ManualSwitch  CurrentSetting=0
  Sum5 : Sum  Inputs=-+|
  Out1 : Outport
  wires:
  Integrator1/1 -> Gain1/1, Manual Switch1/2
  In2/1 -> Sum5/2  "ue"
  Gain4/1 -> Integrator1/1
  Manual Switch1/1 -> Out1/1  "out"
  Sum5/1 -> Gain4/1
  Gain1/1 -> Sum5/1
  Constant/1 -> Manual Switch1/1

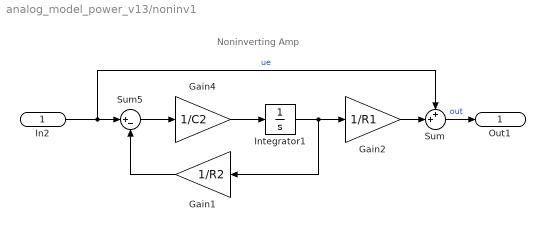
== system analog_model_power_v13/noninv1 ==
  note: Noninverting Amp
  In2 : Inport
  Gain1 : Gain  Gain=1/R2
  Gain2 : Gain  Gain=1/R1
  Gain4 : Gain  Gain=1/C2
  Integrator1 : Integrator
  Sum : Sum  Inputs=++|
  Sum5 : Sum  Inputs=|+-
  Out1 : Outport
  wires:
  Integrator1/1 -> Gain1/1, Gain2/1
  In2/1 -> Sum/1, Sum5/1  "ue"
  Gain4/1 -> Integrator1/1
  Sum/1 -> Out1/1  "out"
  Sum5/1 -> Gain4/1
  Gain1/1 -> Sum5/2
  Gain2/1 -> Sum/2

== matlab function analog_model_power_v13/Subsystem1/MATLAB Function ==
  data: u input; y output
function y = fcn(u)
%#codegen
h=get_param(get_param('analog_model_power_v13/Subsystem1/MATLAB Function','parent'),'handle');
st=get(h,'MaskNames');
sv=get(h,'MaskValues');
s=cell2struct(sv,st,1)
get(h,'MaskValues')

R1=s.R1;
R2=s.R2;
R3=s.R3;
R4=s.R4;
C1=s.C1;

y = R2*(R3+Z4)/(R3*(R1+R2)) * u;
